simulink model "staircase_upanddown_test"  (R2019a)
settings: Solver=VariableStepAuto  StartTime=0.0  StopTime=5000  RelTol=1e-3  EnableMultiTasking=on
StartFcn:
  | clear all
libraries: realtime_pacer_lib x1
settings Model: Creator=johnh  LastModifiedBy=hgarnier
settings DataIOCC: ReturnWorkspaceOutputs=off
settings OptimizationCC: LifeSpan=inf
settings DebuggingCC: PregeneratedLibrarySubsystemCodeDiagnostic=none  SFUnexpectedBacktrackingDiag=warning  SFNoUnconditionalDefaultTransitionDiag=warning  SFExecutionAtInitializationDiag=none  ArithmeticOperatorsInVariantConditions=warning
settings SFSimCC: SimUseLocalCustomCode=off
settings RTWCC: RTWUseLocalCustomCode=off
settings CodeAppCC: StateflowObjectComments=on
settings GRTTargetCC: TargetLangStandard=C89/C90 (ANSI)  GeneratePreprocessorConditionals=Disable all
settings ConfigComp: CovMetricSettings=dw  CovHtmlReporting=on  CovSaveCumulativeToWorkspaceVar=on  CovSaveSingleToWorkspaceVar=on  CovExternalEMLEnable=off

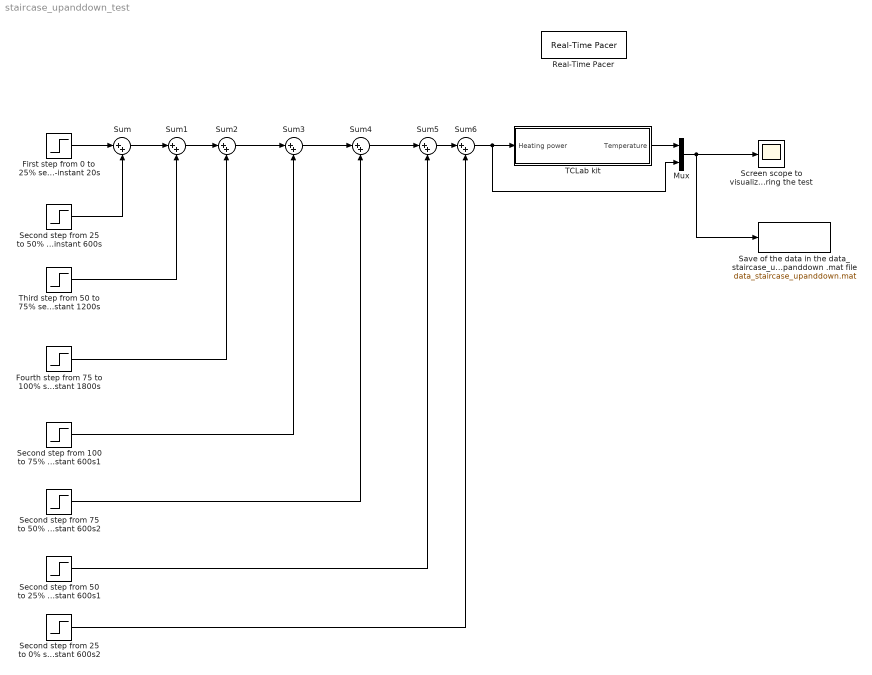
== system staircase_upanddown_test ==
  " Screen scope to visualize the signalsduring the test" : Scope
  First step from 0 to 25% sent at time-instant 20s : Step  Time=20  After=25  SampleTime=0
  Fourth step from 75 to 100% sent at time-instant 1800s : Step  Time=1800  After=25  SampleTime=0
  Mux : Mux  Inputs=2
  Real-Time Pacer : realtime_pacer_lib/Real-Time Pacer  simTimePerRealTime=1
  Save of the data in the data_staircase_upanddown .mat file : ToFile  Filename=data_staircase_upanddown.mat  MatrixName=data0
  Second step from 100 to 75% sent at time-instant 600s1 : Step  Time=2400  After=-25  SampleTime=0
  Second step from 25 to 0% sent at time-instant 600s2 : Step  Time=4200  After=-25  SampleTime=0
  Second step from 25 to 50% sent at time-instant 600s : Step  Time=600  After=25  SampleTime=0
  Second step from 50 to 25% sent at time-instant 600s1 : Step  Time=3600  After=-25  SampleTime=0
  Second step from 75 to 50% sent at time-instant 600s2 : Step  Time=3000  After=-25  SampleTime=0
  Sum{,1..6} (7 alike) : Sum  Inputs=|++
  TCLab kit : Subsystem
  "Third step from 50 to 75% sent at time-instant 1200s " : Step  Time=1200  After=25  SampleTime=0
  wires:
  TCLab kit/1(Temperature) -> Mux/1
  Mux/1 -> Save of the data in the data_staircase_upanddown .mat file/1, " Screen scope to visualize the signalsduring the test"/1
  First step from 0 to 25% sent at time-instant 20s/1 -> Sum/1
  Second step from 25 to 50% sent at time-instant 600s/1 -> Sum/2
  "Third step from 50 to 75% sent at time-instant 1200s "/1 -> Sum1/2
  Fourth step from 75 to 100% sent at time-instant 1800s/1 -> Sum2/2
  Sum/1 -> Sum1/1
  Sum1/1 -> Sum2/1
  Sum2/1 -> Sum3/1
  Sum3/1 -> Sum4/1
  Sum4/1 -> Sum5/1
  Second step from 100 to 75% sent at time-instant 600s1/1 -> Sum3/2
  Second step from 75 to 50% sent at time-instant 600s2/1 -> Sum4/2
  Second step from 50 to 25% sent at time-instant 600s1/1 -> Sum5/2
  Sum5/1 -> Sum6/1
  Sum6/1 -> Mux/2, TCLab kit/1(Heating power)
  Second step from 25 to 0% sent at time-instant 600s2/1 -> Sum6/2

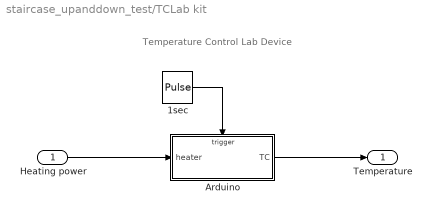
== system staircase_upanddown_test/TCLab kit ==
  note: Temperature Control Lab Device
  Heating power : Inport
  1sec : DiscretePulseGenerator  PulseType=Time based  Period=1  PulseWidth=50
  Arduino : Subsystem  TreatAsAtomicUnit=on
  Temperature : Outport
  wires:
  1sec/1 -> Arduino/Trigger
  Arduino/1(TC) -> Temperature/1
  Heating power/1 -> Arduino/1(heater)

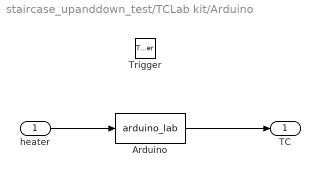
== system staircase_upanddown_test/TCLab kit/Arduino ==
  heater : Inport
  Trigger : TriggerPort  VariantControl=Variant
  Arduino : MATLABFcn  MATLABFcn=arduino_lab
  TC : Outport  InitialOutput=23
  wires:
  heater/1 -> Arduino/1
  Arduino/1 -> TC/1
